simulink subsystem "MODES"  (R2025b)
settings: Solver=VariableStepAuto  StartTime=0.0  StopTime=10.0  RelTol=1e-3
model mask{omgBodSafeTH=0, omgRwDesaturationTH=0, omgRwDesaturationEndTH=0, omgRwMax=0}
  mask prompts: omgBodSafeTH "Body angular velocity Safe mode threshold [rads-1]"; omgRwDesaturationTH "RW angular velocity Desaturation mode threshold [frac of max RW omg]"; omgRwDesaturationEndTH "RW angular velocity Desaturation mode exit threshold [frac of max RW omg]"; omgRwMax "RW maximum angular velocity [rads-1]"
settings Model: Creator=antoniohernandez-rodiciomateos  LastModifiedBy=antoniohernandez-rodiciomateos

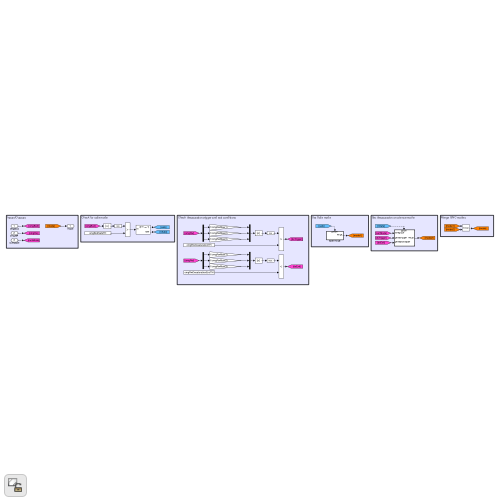
[thumbnail: Simulink's stored preview of the top-level diagram]
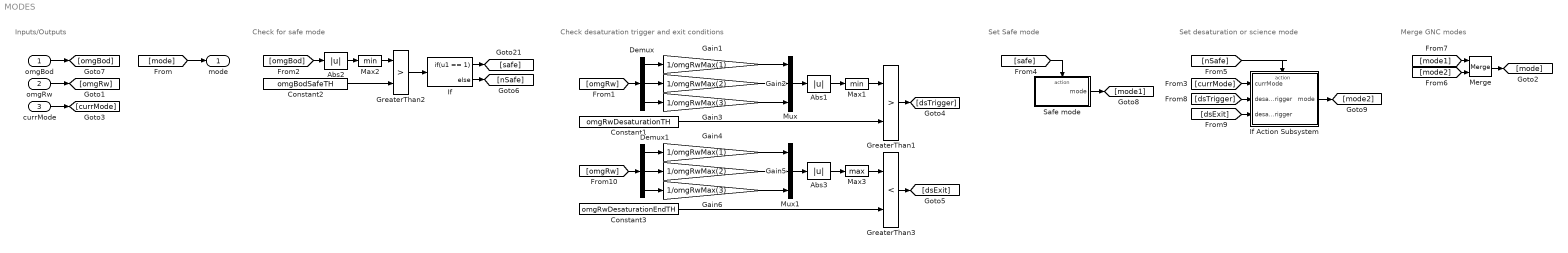
== system MODES ==
  note: Inputs/Outputs
  note: Check for safe mode
  note: Check desaturation trigger and exit conditions
  note: Set Safe mode
  note: Set desaturation or science mode
  note: Merge GNC modes
  omgBod : Inport  PortDimensions=[3 1]
  omgRw : Inport  Port=2  PortDimensions=[3 1]
  currMode : Inport  Port=3  OutDataTypeStr=double  PortDimensions=[1 1]
  Abs1 : Abs  SaturateOnIntegerOverflow=off
  Abs2 : Abs  SaturateOnIntegerOverflow=off
  Abs3 : Abs  SaturateOnIntegerOverflow=off
  Constant1 : Constant  Value=omgRwDesaturationTH
  Constant2 : Constant  Value=omgBodSafeTH
  Constant3 : Constant  Value=omgRwDesaturationEndTH
  Demux : Demux  Outputs=3
  Demux1 : Demux  Outputs=3
  Gain1 : Gain  Gain=1/omgRwMax(1)
  Gain2 : Gain  Gain=1/omgRwMax(2)
  Gain3 : Gain  Gain=1/omgRwMax(3)
  Gain4 : Gain  Gain=1/omgRwMax(1)
  Gain5 : Gain  Gain=1/omgRwMax(2)
  Gain6 : Gain  Gain=1/omgRwMax(3)
  GreaterThan1 : RelationalOperator  Operator=>  OutDataTypeStr=boolean  RndMeth=Simplest  InputSameDT=off
  GreaterThan2 : RelationalOperator  Operator=>  OutDataTypeStr=boolean  RndMeth=Simplest  InputSameDT=off
  GreaterThan3 : RelationalOperator  Operator=<  OutDataTypeStr=boolean  RndMeth=Simplest  InputSameDT=off
  If : If  IfExpression=u1 == 1
  If Action Subsystem : Subsystem  TreatAsAtomicUnit=on
  Max1 : MinMax
  Max2 : MinMax
  Max3 : MinMax  Function=max
  Merge : Merge
  Mux : Mux  Inputs=3
  Mux1 : Mux  Inputs=3
  Safe mode : Subsystem  TreatAsAtomicUnit=on
  mode : Outport  OutDataTypeStr=double  PortDimensions=[1 1]
  wires:
  [mode] -> mode/1
  currMode/1 -> [currMode]
  omgBod/1 -> [omgBod]
  omgRw/1 -> [omgRw]
  Constant2/1 -> GreaterThan2/2
  Abs2/1 -> Max2/1
  If/1 -> [safe]
  [omgBod] -> Abs2/1
  If/2 -> [nSafe]
  Max2/1 -> GreaterThan2/1
  GreaterThan2/1 -> If/1
  Gain1/1 -> Mux/1
  Abs1/1 -> Max1/1
  [omgRw] -> Demux1/1
  Gain6/1 -> Mux1/3
  Mux/1 -> Abs1/1
  Constant3/1 -> GreaterThan3/2
  Abs3/1 -> Max3/1
  Demux1/1 -> Gain4/1
  Demux/1 -> Gain1/1
  Gain3/1 -> Mux/3
  Demux/2 -> Gain2/1
  Mux1/1 -> Abs3/1
  GreaterThan1/1 -> [dsTrigger]
  Demux1/3 -> Gain6/1
  Gain4/1 -> Mux1/1
  Max3/1 -> GreaterThan3/1
  GreaterThan3/1 -> [dsExit]
  Constant1/1 -> GreaterThan1/2
  Gain5/1 -> Mux1/2
  Demux/3 -> Gain3/1
  Max1/1 -> GreaterThan1/1
  Gain2/1 -> Mux/2
  Demux1/2 -> Gain5/1
  [omgRw] -> Demux/1
  [currMode] -> If Action Subsystem/1(currMode)
  If Action Subsystem/1(mode) -> [mode2]
  [dsExit] -> If Action Subsystem/3(desatExitTrigger)
  [dsTrigger] -> If Action Subsystem/2(desatTrigger)
  [safe] -> Safe mode/Action
  Safe mode/1(mode) -> [mode1]
  [nSafe] -> If Action Subsystem/Action
  [mode1] -> Merge/1
  [mode2] -> Merge/2
  Merge/1 -> [mode]

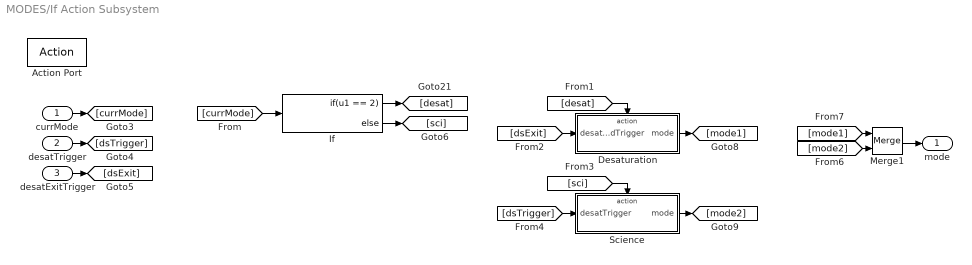
== system MODES/If Action Subsystem ==
  currMode : Inport  OutDataTypeStr=double  PortDimensions=[1 1]
  desatTrigger : Inport  Port=2  OutDataTypeStr=boolean  PortDimensions=[1 1]
  desatExitTrigger : Inport  Port=3  OutDataTypeStr=boolean  PortDimensions=[1 1]
  Action Port : ActionPort
  Desaturation : Subsystem  TreatAsAtomicUnit=on
  If : If  IfExpression=u1 == 2
  Merge1 : Merge
  Science : Subsystem  TreatAsAtomicUnit=on
  mode : Outport  OutDataTypeStr=double  PortDimensions=[1 1]
  wires:
  currMode/1 -> [currMode]
  desatExitTrigger/1 -> [dsExit]
  desatTrigger/1 -> [dsTrigger]
  [currMode] -> If/1
  If/2 -> [sci]
  If/1 -> [desat]
  Desaturation/1(mode) -> [mode1]
  [mode1] -> Merge1/1
  [sci] -> Science/Action
  [dsTrigger] -> Science/1(desatTrigger)
  Science/1(mode) -> [mode2]
  [mode2] -> Merge1/2
  [dsExit] -> Desaturation/1(desatEndTrigger)
  [desat] -> Desaturation/Action
  Merge1/1 -> mode/1

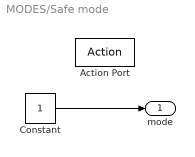
== system MODES/Safe mode ==
  Action Port : ActionPort
  Constant : Constant
  mode : Outport  OutDataTypeStr=double  PortDimensions=[1 1]
  wires:
  Constant/1 -> mode/1

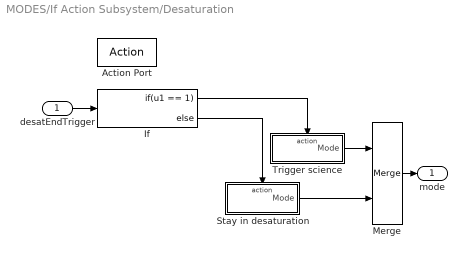
== system MODES/If Action Subsystem/Desaturation ==
  desatEndTrigger : Inport  OutDataTypeStr=boolean  PortDimensions=[1 1]
  Action Port : ActionPort
  If : If  IfExpression=u1 == 1
  Merge : Merge
  Stay in desaturation : Subsystem  TreatAsAtomicUnit=on
  Trigger science : Subsystem  TreatAsAtomicUnit=on
  mode : Outport  OutDataTypeStr=double  PortDimensions=[1 1]
  wires:
  Stay in desaturation/1(Mode) -> Merge/2
  Trigger science/1(Mode) -> Merge/1
  Merge/1 -> mode/1
  If/2 -> Stay in desaturation/Action
  If/1 -> Trigger science/Action
  desatEndTrigger/1 -> If/1

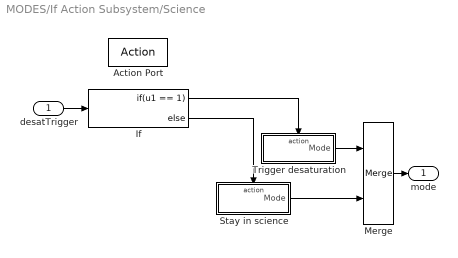
== system MODES/If Action Subsystem/Science ==
  desatTrigger : Inport  OutDataTypeStr=boolean  PortDimensions=[1 1]
  Action Port : ActionPort
  If : If  IfExpression=u1 == 1
  Merge : Merge
  Stay in science : Subsystem  TreatAsAtomicUnit=on
  Trigger desaturation : Subsystem  TreatAsAtomicUnit=on
  mode : Outport  OutDataTypeStr=double  PortDimensions=[1 1]
  wires:
  If/2 -> Stay in science/Action
  Merge/1 -> mode/1
  Stay in science/1(Mode) -> Merge/2
  desatTrigger/1 -> If/1
  Trigger desaturation/1(Mode) -> Merge/1
  If/1 -> Trigger desaturation/Action

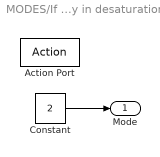
== system MODES/If Action Subsystem/Desaturation/Stay in desaturation ==
  Action Port : ActionPort
  Constant : Constant  Value=2
  Mode : Outport  OutDataTypeStr=double  PortDimensions=[1 1]
  wires:
  Constant/1 -> Mode/1

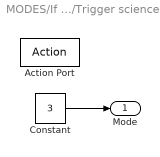
== system MODES/If Action Subsystem/Desaturation/Trigger science ==
  Action Port : ActionPort
  Constant : Constant  Value=3
  Mode : Outport  OutDataTypeStr=double  PortDimensions=[1 1]
  wires:
  Constant/1 -> Mode/1

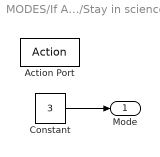
== system MODES/If Action Subsystem/Science/Stay in science ==
  Action Port : ActionPort
  Constant : Constant  Value=3
  Mode : Outport  OutDataTypeStr=double  PortDimensions=[1 1]
  wires:
  Constant/1 -> Mode/1

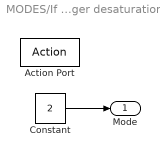
== system MODES/If Action Subsystem/Science/Trigger desaturation ==
  Action Port : ActionPort
  Constant : Constant  Value=2
  Mode : Outport  OutDataTypeStr=double  PortDimensions=[1 1]
  wires:
  Constant/1 -> Mode/1
